simulink model "screening_stage2_review"  (R2026a)
settings: Solver=VariableStepAuto
values from neighbouring files (symbols this model uses):
  m = result.lesionMasks.(code)    [runScreeningPipeline.m]
undefined symbols (not defined in the file or in its folder): n
settings Model: Creator=keert  LastModifiedBy=keert

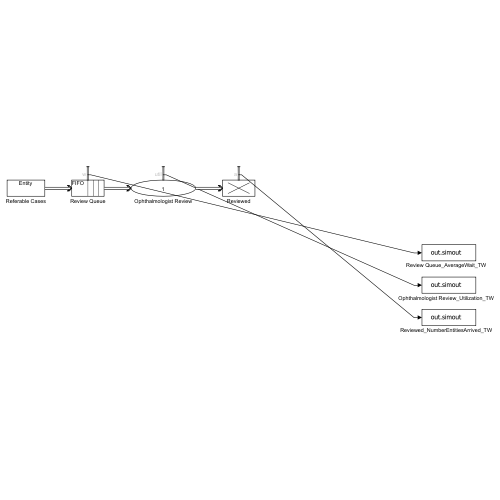
[thumbnail: Simulink's stored preview of the top-level diagram]
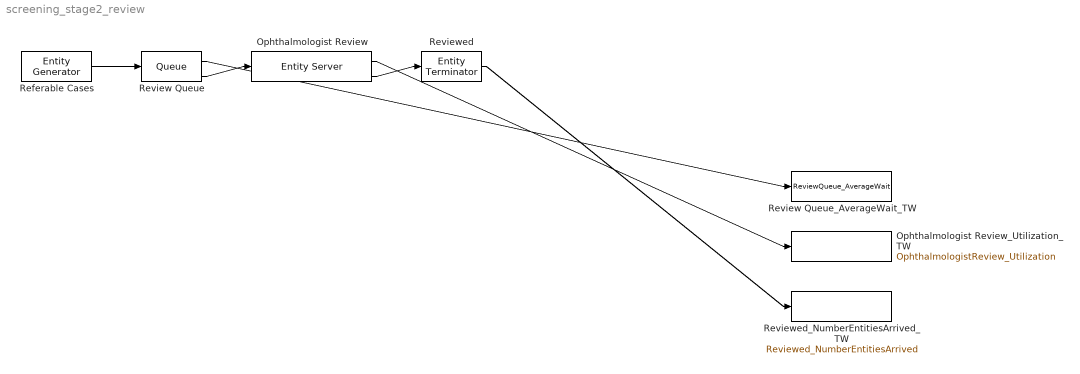
== system screening_stage2_review ==
  Ophthalmologist Review : EntityServer  InputPortMessageModes=m  OutputPortMessageModes=n,m  Capacity=1  ServiceTimeValue=30  Utilization=on
      settings: OutputPortMap=o5,o9
  Ophthalmologist Review_Utilization_TW : ToWorkspace  VariableName=OphthalmologistReview_Utilization  SaveFormat=Structure  SampleTime=-1
  Referable Cases : EntityGenerator  OutputPortMessageModes=m  Period=262.7737  EntityType=Structured  EntityTypeName=Entity
  Review Queue : Queue  InputPortMessageModes=m  OutputPortMessageModes=n,m  AverageWait=on
      settings: OutputPortMap=o2,o5
  Review Queue_AverageWait_TW : ToWorkspace  VariableName=ReviewQueue_AverageWait  SaveFormat=Structure  SampleTime=-1
  Reviewed : EntityTerminator  InputPortMessageModes=m  NumberEntitiesArrived=on
      settings: OutputPortMap=o0
  Reviewed_NumberEntitiesArrived_TW : ToWorkspace  VariableName=Reviewed_NumberEntitiesArrived  SaveFormat=Structure  SampleTime=-1
  wires:
  Review Queue/1 -> Review Queue_AverageWait_TW/1
  Ophthalmologist Review/1 -> Ophthalmologist Review_Utilization_TW/1
  Reviewed/1 -> Reviewed_NumberEntitiesArrived_TW/1
  Referable Cases/1 -> Review Queue/1
  Review Queue/2 -> Ophthalmologist Review/1
  Ophthalmologist Review/2 -> Reviewed/1
